simulink model "LundellAlternatorAC"  (R2018a)
settings: Solver=VariableStepAuto  StartTime=0  StopTime=0.2  FixedStep=1e-6
undefined symbols (not defined in the file): alternator, i_f, n_r, r_l
libraries: fl_lib x28, nesl_utility x27, powerlib_meascontrol x6, elec_lib x6, SimscapeCustomBlocks_lib x2
settings Model: Creator=gabrielrodrigues  LastModifiedBy=gabrielrodrigues
settings DataIOCC: ReturnWorkspaceOutputs=on
settings CodeAppCC: StateflowObjectComments=on
settings SimscapeCC: SimscapeNormalizeSystem=off  SimscapeLogType=local  SimscapeLogLimitData=off

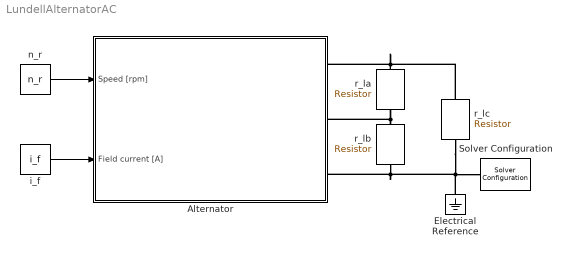
== system LundellAlternatorAC ==
  Alternator : Subsystem
  Electrical Reference : fl_lib/Electrical/Electrical Elements/Electrical Reference
  Solver Configuration : nesl_utility/Solver Configuration  PhysicalDomain=network_engine_domain  SubClassName=solver  LeftPortType=input  RightPortType=generic  Tones=[]  Harmonics=[]  SimulateNoise=off  Profile=off  UseLocalSampling=off  EnableSwitchedLinearOptims=on  FrequencyDomain=off  UseCCode=off  RelTol=0.001  AbsTol=1e-06  MinStep=1e-09  ToWorkspace=off  RevertToSquareIcSolve=off  NumHomotopyIterations=100  PhasorMode=off  PhasorModeNumHarmonics=1  DoDC=off  ResidualTolerance=1e-09  UseLocalSolver=on  LocalSolverChoice=NE_TRAPEZOIDAL_ADVANCER  LocalSolverSampleTime=1e-06  DoFixedCost=on  MaxNonlinIter=20  MaxModeIter=2  LinearAlgebra=Sparse  EquationFormulation=NE_TIME_EF  DelaysMemoryBudget=1024  AutomaticFiltering=on  FilteringTimeConstant=0.001
  i_f : Constant  Value=i_f
  n_r : Constant  Value=n_r
  r_la : fl_lib/Electrical/Electrical Elements/Resistor  R=r_l Ohm  i_specify=off  i_priority=None  i=0 A  i_nominal_specify=off  i_nominal_unit=A  i_nominal_value=1  v_specify=off  v_priority=None  v=0 V  v_nominal_specify=off  v_nominal_unit=V  v_nominal_value=1
  r_lb : fl_lib/Electrical/Electrical Elements/Resistor  R=r_l Ohm  i_specify=off  i_priority=None  i=0 A  i_nominal_specify=off  i_nominal_unit=A  i_nominal_value=1  v_specify=off  v_priority=None  v=0 V  v_nominal_specify=off  v_nominal_unit=V  v_nominal_value=1
  r_lc : fl_lib/Electrical/Electrical Elements/Resistor  R=r_l Ohm  i_specify=off  i_priority=None  i=0 A  i_nominal_specify=off  i_nominal_unit=A  i_nominal_value=1  v_specify=off  v_priority=None  v=0 V  v_nominal_specify=off  v_nominal_unit=V  v_nominal_value=1
  wires:
  n_r/1 -> Alternator/1(Speed [rpm])
  i_f/1 -> Alternator/2(Field current [A])
  connections:
  r_la/RConn1 -- r_lb/LConn1 -- Alternator/RConn2
  Electrical Reference/LConn1 -- Solver Configuration/RConn1 -- Alternator/RConn3 -- r_lb/RConn1 -- r_lc/LConn1
  r_la/LConn1 -- r_lc/RConn1 -- Alternator/RConn1

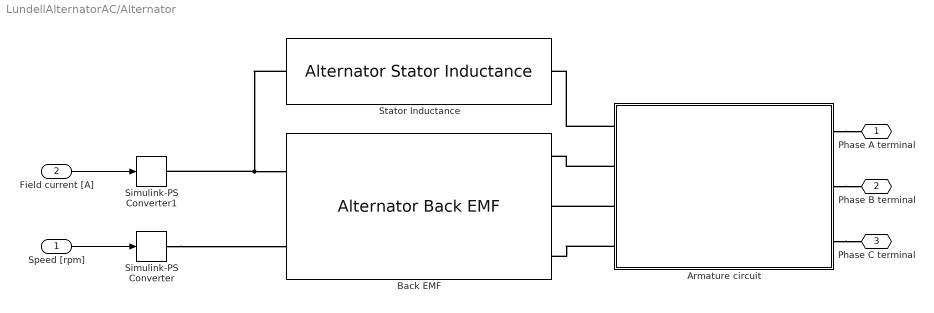
== system LundellAlternatorAC/Alternator ==
  Speed [rpm] : Inport
  Field current [A] : Inport  Port=2
  Armature circuit : Subsystem  Variant=on
  Back EMF : SimscapeCustomBlocks_lib/Alternator/Alternator Back EMF  p=alternator.p  omega_r_specify=off  omega_r_priority=None  omega_r=0 rad/s  omega_r_nominal_specify=off  omega_r_nominal_unit=rad/s  omega_r_nominal_value=1  omega_e_specify=off  omega_e_priority=None  omega_e=0 rad/s  omega_e_nominal_specify=off  omega_e_nominal_unit=rad/s  omega_e_nominal_value=1  theta_e_specify=off  theta_e_priority=None  theta_e=0 rad  theta_e_nominal_specify=off  theta_e_nominal_unit=rad  theta_e_nominal_value=1  k_e_specify=off  k_e_priority=None  k_e=0 s*V/rad/A  k_e_nominal_specify=off  k_e_nominal_unit=s*V/rad/A  k_e_nominal_value=1  e_specify=off  e_priority=None  e=0 rpm  e_nominal_specify=off  e_nominal_unit=rpm  e_nominal_value=1
  Simulink-PS Converter : nesl_utility/Simulink-PS Converter  PhysicalDomain=network_engine_domain  SubClassName=ps_input  LeftPortType=input  RightPortType=output  PseudoPeriodic=off  Frequencies=[]  NoiseDistribution=none  NoiseParameters=[]  Unit=1  AffineConversion=off  FilteringAndDerivatives=provide  SimscapeFilterOrder=1  InputFilterTimeConstant=0.001  UdotUserProvided=0
  Simulink-PS Converter1 : nesl_utility/Simulink-PS Converter  PhysicalDomain=network_engine_domain  SubClassName=ps_input  LeftPortType=input  RightPortType=output  PseudoPeriodic=off  Frequencies=[]  NoiseDistribution=none  NoiseParameters=[]  Unit=1  AffineConversion=off  FilteringAndDerivatives=provide  SimscapeFilterOrder=1  InputFilterTimeConstant=0.001  UdotUserProvided=0
  Stator Inductance : SimscapeCustomBlocks_lib/Alternator/Alternator Stator Inductance
  Phase A terminal : PMIOPort  Side=Right
  Phase B terminal : PMIOPort  Port=2  Side=Right
  Phase C terminal : PMIOPort  Port=3  Side=Right
  wires:
  Speed [rpm]/1 -> Simulink-PS Converter/1
  Field current [A]/1 -> Simulink-PS Converter1/1
  connections:
  Armature circuit/RConn1 -- Phase A terminal/RConn1
  Armature circuit/RConn2 -- Phase B terminal/RConn1
  Armature circuit/RConn3 -- Phase C terminal/RConn1
  Armature circuit/LConn3 -- Back EMF/RConn2
  Armature circuit/LConn2 -- Back EMF/RConn1
  Armature circuit/LConn4 -- Back EMF/RConn3
  Simulink-PS Converter/RConn1 -- Back EMF/LConn2
  Armature circuit/LConn1 -- Stator Inductance/RConn1
  Stator Inductance/LConn1 -- Simulink-PS Converter1/RConn1 -- Back EMF/LConn1

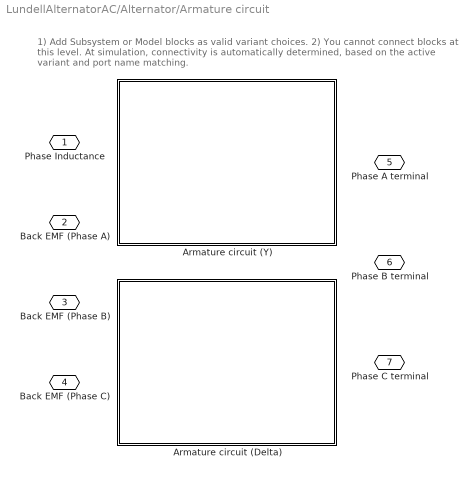
== system LundellAlternatorAC/Alternator/Armature circuit ==
  note: 1) Add Subsystem or Model blocks as valid variant choices.
      | 2) You cannot connect blocks at this level. At simulation, connectivity is automatically
      | determined, based on the active variant and port name matching.
  Armature circuit (Delta) : Subsystem  VariantControl=deltaStatorConnection
  Armature circuit (Y) : Subsystem  VariantControl=yStatorConnection
  Phase Inductance : PMIOPort  Side=Left
  Back EMF (Phase A) : PMIOPort  Port=2  Side=Left
  Back EMF (Phase B) : PMIOPort  Port=3  Side=Left
  Back EMF (Phase C) : PMIOPort  Port=4  Side=Left
  Phase A terminal : PMIOPort  Port=5  Side=Right
  Phase B terminal : PMIOPort  Port=6  Side=Right
  Phase C terminal : PMIOPort  Port=7  Side=Right

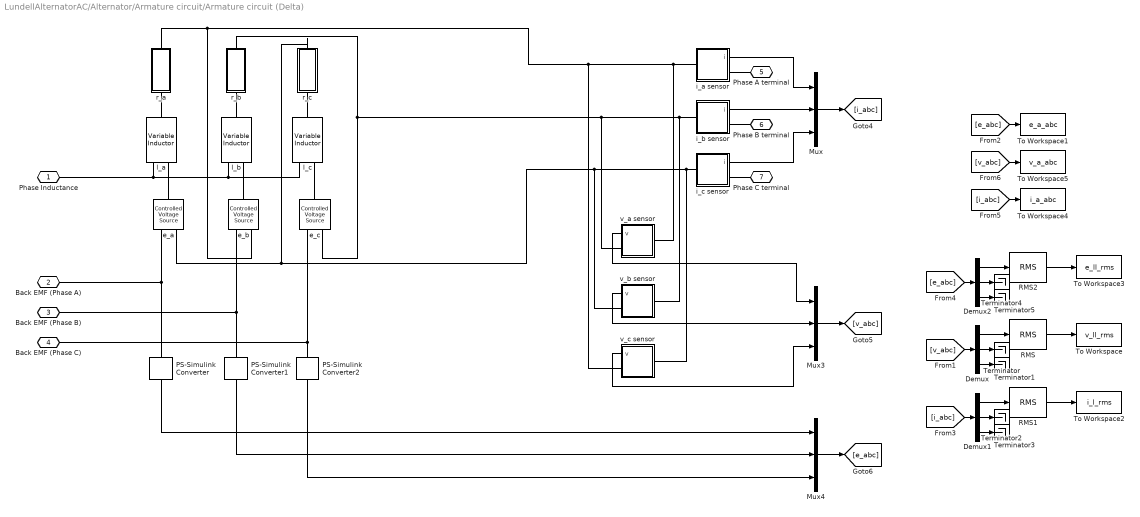
== system LundellAlternatorAC/Alternator/Armature circuit/Armature circuit (Delta) ==
  Demux : Demux  Outputs=3
  Demux1 : Demux  Outputs=3
  Demux2 : Demux  Outputs=3
  Mux : Mux  Inputs=3
  Mux3 : Mux  Inputs=3
  Mux4 : Mux  Inputs=3
  PS-Simulink Converter : nesl_utility/PS-Simulink Converter  PhysicalDomain=network_engine_domain  SubClassName=ps_output  LeftPortType=input  RightPortType=output  PseudoPeriodic=off  Frequencies=[]  Unit=1  AffineConversion=off
  PS-Simulink Converter1 : nesl_utility/PS-Simulink Converter  PhysicalDomain=network_engine_domain  SubClassName=ps_output  LeftPortType=input  RightPortType=output  PseudoPeriodic=off  Frequencies=[]  Unit=1  AffineConversion=off
  PS-Simulink Converter2 : nesl_utility/PS-Simulink Converter  PhysicalDomain=network_engine_domain  SubClassName=ps_output  LeftPortType=input  RightPortType=output  PseudoPeriodic=off  Frequencies=[]  Unit=1  AffineConversion=off
  RMS : powerlib_meascontrol/Measurements/RMS  TrueRMS=on  Freq=8*2000/60  RMSInit=120  Ts=0
      settings: SourceProductName=Simscape Electrical
  RMS1 : powerlib_meascontrol/Measurements/RMS  TrueRMS=on  Freq=8*2000/60  RMSInit=120  Ts=0
      settings: SourceProductName=Simscape Electrical
  RMS2 : powerlib_meascontrol/Measurements/RMS  TrueRMS=on  Freq=8*2000/60  RMSInit=120  Ts=0
      settings: SourceProductName=Simscape Electrical
  Terminator{,1..5} (6 alike) : Terminator
  To Workspace : ToWorkspace  VariableName=v_ll_rms  SaveFormat=Timeseries  SampleTime=-1
  To Workspace1 : ToWorkspace  VariableName=e_a_abc  SaveFormat=Timeseries  SampleTime=-1
  To Workspace2 : ToWorkspace  VariableName=i_l_rms  SaveFormat=Timeseries  SampleTime=-1
  To Workspace3 : ToWorkspace  VariableName=e_ll_rms  SaveFormat=Timeseries  SampleTime=-1
  To Workspace4 : ToWorkspace  VariableName=i_a_abc  SaveFormat=Timeseries  SampleTime=-1
  To Workspace5 : ToWorkspace  VariableName=v_a_abc  SaveFormat=Timeseries  SampleTime=-1
  e_a : fl_lib/Electrical/Electrical Sources/Controlled Voltage Source
  e_b : fl_lib/Electrical/Electrical Sources/Controlled Voltage Source
  e_c : fl_lib/Electrical/Electrical Sources/Controlled Voltage Source
  i_a sensor : Subsystem
  i_b sensor : Subsystem
  i_c sensor : Subsystem
  l_a : elec_lib/Passive Devices/Variable Inductor  prm=1  Lmin=1e-6 H  g=1e-9 1/Ohm  i0=0 A  phi0=0 Wb
      settings: SourceProductName=Simscape Electronics  SourceProductBaseCode=SN
  l_b : elec_lib/Passive Devices/Variable Inductor  prm=1  Lmin=1e-6 H  g=1e-9 1/Ohm  i0=0 A  phi0=0 Wb
      settings: SourceProductName=Simscape Electronics  SourceProductBaseCode=SN
  l_c : elec_lib/Passive Devices/Variable Inductor  prm=1  Lmin=1e-6 H  g=1e-9 1/Ohm  i0=0 A  phi0=0 Wb
      settings: SourceProductName=Simscape Electronics  SourceProductBaseCode=SN
  r_a : Subsystem  mask{r_ref=alternator.stator.r.value, T_ref=alternator.stator.r.T_ref, T=alternator.stator.r.T, alpha=alternator.stator.r.alpha}
      mask prompts: r_ref "Nominal resistance [Ohm]"; T_ref "Reference temperature [oC]"; T "Resistor temperature [oC]"; alpha "Temperature Coefficient [1/oC]"
  r_b : Subsystem  mask{r_ref=alternator.stator.r.value, T_ref=alternator.stator.r.T_ref, T=alternator.stator.r.T, alpha=alternator.stator.r.alpha}
      mask prompts: r_ref "Nominal resistance [Ohm]"; T_ref "Reference temperature [oC]"; T "Resistor temperature [oC]"; alpha "Temperature Coefficient [1/oC]"
  r_c : Subsystem  mask{r_ref=alternator.stator.r.value, T_ref=alternator.stator.r.T_ref, T=alternator.stator.r.T, alpha=alternator.stator.r.alpha}
      mask prompts: r_ref "Nominal resistance [Ohm]"; T_ref "Reference temperature [oC]"; T "Resistor temperature [oC]"; alpha "Temperature Coefficient [1/oC]"
  v_a sensor : Subsystem
  v_b sensor : Subsystem
  v_c sensor : Subsystem
  Phase Inductance : PMIOPort  Side=Left
  Back EMF (Phase A) : PMIOPort  Port=2  Side=Left
  Back EMF (Phase B) : PMIOPort  Port=3  Side=Left
  Back EMF (Phase C) : PMIOPort  Port=4  Side=Left
  Phase A terminal : PMIOPort  Port=5  Side=Right
  Phase B terminal : PMIOPort  Port=6  Side=Right
  Phase C terminal : PMIOPort  Port=7  Side=Right
  wires:
  i_a sensor/1(i) -> Mux/1
  i_b sensor/1(i) -> Mux/2
  i_c sensor/1(i) -> Mux/3
  Mux/1 -> [i_abc]
  Mux3/1 -> [v_abc]
  v_b sensor/1(v) -> Mux3/2
  v_c sensor/1(v) -> Mux3/3
  v_a sensor/1(v) -> Mux3/1
  PS-Simulink Converter/1 -> Mux4/1
  PS-Simulink Converter1/1 -> Mux4/2
  PS-Simulink Converter2/1 -> Mux4/3
  Mux4/1 -> [e_abc]
  Demux/3 -> Terminator1/1
  Demux/2 -> Terminator/1
  Demux2/2 -> Terminator4/1
  [e_abc] -> Demux2/1
  RMS2/1 -> To Workspace3/1
  Demux2/1 -> RMS2/1
  Demux2/3 -> Terminator5/1
  Demux1/2 -> Terminator2/1
  [e_abc] -> To Workspace1/1
  RMS/1 -> To Workspace/1
  Demux/1 -> RMS/1
  RMS1/1 -> To Workspace2/1
  [i_abc] -> Demux1/1
  [v_abc] -> Demux/1
  Demux1/3 -> Terminator3/1
  [v_abc] -> To Workspace5/1
  Demux1/1 -> RMS1/1
  [i_abc] -> To Workspace4/1
  connections:
  i_a sensor/RConn1 -- Phase A terminal/RConn1
  Back EMF (Phase A)/RConn1 -- e_a/RConn1 -- PS-Simulink Converter/LConn1
  Back EMF (Phase B)/RConn1 -- e_b/RConn1 -- PS-Simulink Converter1/LConn1
  Back EMF (Phase C)/RConn1 -- e_c/RConn1 -- PS-Simulink Converter2/LConn1
  e_c/LConn1 -- l_c/LConn2
  e_b/LConn1 -- l_b/LConn2
  e_a/LConn1 -- l_a/LConn2
  r_c/LConn1 -- l_c/RConn1
  r_b/LConn1 -- l_b/RConn1
  r_a/LConn1 -- l_a/RConn1
  i_c sensor/RConn1 -- Phase C terminal/RConn1
  i_b sensor/RConn1 -- Phase B terminal/RConn1
  l_a/LConn1 -- Phase Inductance/RConn1 -- l_b/LConn1 -- l_c/LConn1
  e_b/RConn2 -- v_a sensor/LConn1 -- i_a sensor/LConn1 -- v_c sensor/RConn1 -- r_a/RConn1
  v_a sensor/RConn1 -- i_b sensor/LConn1 -- v_b sensor/LConn1 -- e_c/RConn2 -- r_b/RConn1
  e_a/RConn2 -- v_c sensor/LConn1 -- i_c sensor/LConn1 -- v_b sensor/RConn1 -- r_c/RConn1

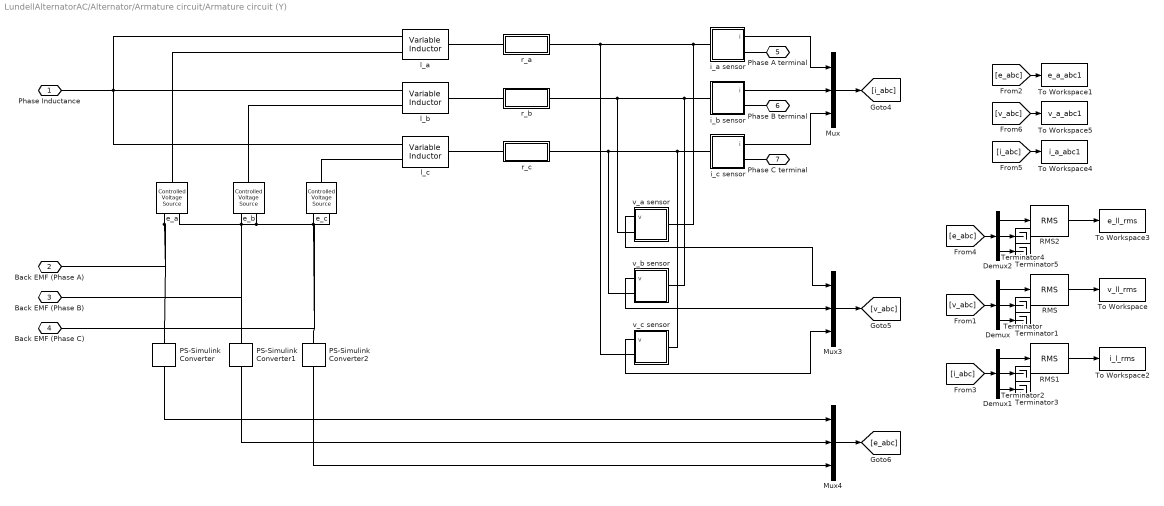
== system LundellAlternatorAC/Alternator/Armature circuit/Armature circuit (Y) ==
  Demux : Demux  Outputs=3
  Demux1 : Demux  Outputs=3
  Demux2 : Demux  Outputs=3
  Mux : Mux  Inputs=3
  Mux3 : Mux  Inputs=3
  Mux4 : Mux  Inputs=3
  PS-Simulink Converter : nesl_utility/PS-Simulink Converter  PhysicalDomain=network_engine_domain  SubClassName=ps_output  LeftPortType=input  RightPortType=output  PseudoPeriodic=off  Frequencies=[]  Unit=1  AffineConversion=off
  PS-Simulink Converter1 : nesl_utility/PS-Simulink Converter  PhysicalDomain=network_engine_domain  SubClassName=ps_output  LeftPortType=input  RightPortType=output  PseudoPeriodic=off  Frequencies=[]  Unit=1  AffineConversion=off
  PS-Simulink Converter2 : nesl_utility/PS-Simulink Converter  PhysicalDomain=network_engine_domain  SubClassName=ps_output  LeftPortType=input  RightPortType=output  PseudoPeriodic=off  Frequencies=[]  Unit=1  AffineConversion=off
  RMS : powerlib_meascontrol/Measurements/RMS  TrueRMS=on  Freq=8*2000/60  RMSInit=120  Ts=0
      settings: SourceProductName=Simscape Electrical
  RMS1 : powerlib_meascontrol/Measurements/RMS  TrueRMS=on  Freq=8*2000/60  RMSInit=120  Ts=0
      settings: SourceProductName=Simscape Electrical
  RMS2 : powerlib_meascontrol/Measurements/RMS  TrueRMS=on  Freq=8*2000/60  RMSInit=120  Ts=0
      settings: SourceProductName=Simscape Electrical
  Terminator{,1..5} (6 alike) : Terminator
  To Workspace : ToWorkspace  VariableName=v_ll_rms  SaveFormat=Timeseries  SampleTime=-1
  To Workspace1 : ToWorkspace  VariableName=e_a_abc1  SaveFormat=Timeseries  SampleTime=-1
  To Workspace2 : ToWorkspace  VariableName=i_l_rms  SaveFormat=Timeseries  SampleTime=-1
  To Workspace3 : ToWorkspace  VariableName=e_ll_rms  SaveFormat=Timeseries  SampleTime=-1
  To Workspace4 : ToWorkspace  VariableName=i_a_abc1  SaveFormat=Timeseries  SampleTime=-1
  To Workspace5 : ToWorkspace  VariableName=v_a_abc1  SaveFormat=Timeseries  SampleTime=-1
  e_a : fl_lib/Electrical/Electrical Sources/Controlled Voltage Source
  e_b : fl_lib/Electrical/Electrical Sources/Controlled Voltage Source
  e_c : fl_lib/Electrical/Electrical Sources/Controlled Voltage Source
  i_a sensor : Subsystem
  i_b sensor : Subsystem
  i_c sensor : Subsystem
  l_a : elec_lib/Passive Devices/Variable Inductor  prm=1  Lmin=1e-6 H  g=1e-9 1/Ohm  i0=0 A  phi0=0 Wb
      settings: SourceProductName=Simscape Electronics  SourceProductBaseCode=SN
  l_b : elec_lib/Passive Devices/Variable Inductor  prm=1  Lmin=1e-6 H  g=1e-9 1/Ohm  i0=0 A  phi0=0 Wb
      settings: SourceProductName=Simscape Electronics  SourceProductBaseCode=SN
  l_c : elec_lib/Passive Devices/Variable Inductor  prm=1  Lmin=1e-6 H  g=1e-9 1/Ohm  i0=0 A  phi0=0 Wb
      settings: SourceProductName=Simscape Electronics  SourceProductBaseCode=SN
  r_a : Subsystem  mask{r_ref=alternator.stator.r.value, T_ref=alternator.stator.r.T_ref, T=alternator.stator.r.T, alpha=alternator.stator.r.alpha}
      mask prompts: r_ref "Nominal resistance [Ohm]"; T_ref "Reference temperature [oC]"; T "Resistor temperature [oC]"; alpha "Temperature Coefficient [1/oC]"
  r_b : Subsystem  mask{r_ref=alternator.stator.r.value, T_ref=alternator.stator.r.T_ref, T=alternator.stator.r.T, alpha=alternator.stator.r.alpha}
      mask prompts: r_ref "Nominal resistance [Ohm]"; T_ref "Reference temperature [oC]"; T "Resistor temperature [oC]"; alpha "Temperature Coefficient [1/oC]"
  r_c : Subsystem  mask{r_ref=alternator.stator.r.value, T_ref=alternator.stator.r.T_ref, T=alternator.stator.r.T, alpha=alternator.stator.r.alpha}
      mask prompts: r_ref "Nominal resistance [Ohm]"; T_ref "Reference temperature [oC]"; T "Resistor temperature [oC]"; alpha "Temperature Coefficient [1/oC]"
  v_a sensor : Subsystem
  v_b sensor : Subsystem
  v_c sensor : Subsystem
  Phase Inductance : PMIOPort  Side=Left
  Back EMF (Phase A) : PMIOPort  Port=2  Side=Left
  Back EMF (Phase B) : PMIOPort  Port=3  Side=Left
  Back EMF (Phase C) : PMIOPort  Port=4  Side=Left
  Phase A terminal : PMIOPort  Port=5  Side=Right
  Phase B terminal : PMIOPort  Port=6  Side=Right
  Phase C terminal : PMIOPort  Port=7  Side=Right
  wires:
  i_a sensor/1(i) -> Mux/1
  i_b sensor/1(i) -> Mux/2
  i_c sensor/1(i) -> Mux/3
  Mux/1 -> [i_abc]
  Mux3/1 -> [v_abc]
  v_b sensor/1(v) -> Mux3/2
  v_c sensor/1(v) -> Mux3/3
  v_a sensor/1(v) -> Mux3/1
  PS-Simulink Converter/1 -> Mux4/1
  PS-Simulink Converter1/1 -> Mux4/2
  PS-Simulink Converter2/1 -> Mux4/3
  Mux4/1 -> [e_abc]
  Demux/3 -> Terminator1/1
  Demux/2 -> Terminator/1
  Demux2/2 -> Terminator4/1
  [e_abc] -> Demux2/1
  RMS2/1 -> To Workspace3/1
  Demux2/1 -> RMS2/1
  Demux2/3 -> Terminator5/1
  Demux1/2 -> Terminator2/1
  [e_abc] -> To Workspace1/1
  RMS/1 -> To Workspace/1
  Demux/1 -> RMS/1
  RMS1/1 -> To Workspace2/1
  [i_abc] -> Demux1/1
  [v_abc] -> Demux/1
  Demux1/3 -> Terminator3/1
  [v_abc] -> To Workspace5/1
  Demux1/1 -> RMS1/1
  [i_abc] -> To Workspace4/1
  connections:
  i_a sensor/RConn1 -- Phase A terminal/RConn1
  e_a/RConn2 -- e_c/RConn2 -- e_b/RConn2
  e_c/LConn1 -- l_c/LConn2
  e_b/LConn1 -- l_b/LConn2
  e_a/LConn1 -- l_a/LConn2
  r_c/LConn1 -- l_c/RConn1
  r_b/LConn1 -- l_b/RConn1
  r_a/LConn1 -- l_a/RConn1
  i_a sensor/LConn1 -- v_a sensor/LConn1 -- v_c sensor/RConn1 -- r_a/RConn1
  i_c sensor/RConn1 -- Phase C terminal/RConn1
  i_b sensor/RConn1 -- Phase B terminal/RConn1
  i_c sensor/LConn1 -- v_c sensor/LConn1 -- v_b sensor/RConn1 -- r_c/RConn1
  v_a sensor/RConn1 -- v_b sensor/LConn1 -- i_b sensor/LConn1 -- r_b/RConn1
  l_a/LConn1 -- Phase Inductance/RConn1 -- l_c/LConn1 -- l_b/LConn1
  e_a/RConn1 -- Back EMF (Phase A)/RConn1 -- PS-Simulink Converter/LConn1
  e_b/RConn1 -- Back EMF (Phase B)/RConn1 -- PS-Simulink Converter1/LConn1
  e_c/RConn1 -- Back EMF (Phase C)/RConn1 -- PS-Simulink Converter2/LConn1

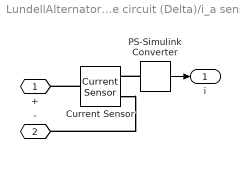
== system LundellAlternatorAC/Alternator/Armature circuit/Armature circuit (Delta)/i_a sensor ==
  Current Sensor : fl_lib/Electrical/Electrical Sensors/Current Sensor
  PS-Simulink Converter : nesl_utility/PS-Simulink Converter  PhysicalDomain=network_engine_domain  SubClassName=ps_output  LeftPortType=input  RightPortType=output  PseudoPeriodic=off  Frequencies=[]  Unit=1  AffineConversion=off
  + : PMIOPort  Side=Left
  - : PMIOPort  Port=2  Side=Right
  i : Outport
  wires:
  PS-Simulink Converter/1 -> i/1
  connections:
  Current Sensor/RConn2 -- -/RConn1
  Current Sensor/LConn1 -- +/RConn1
  PS-Simulink Converter/LConn1 -- Current Sensor/RConn1

== system LundellAlternatorAC/Alternator/Armature circuit/Armature circuit (Delta)/i_b sensor ==
  Current Sensor : fl_lib/Electrical/Electrical Sensors/Current Sensor
  PS-Simulink Converter : nesl_utility/PS-Simulink Converter  PhysicalDomain=network_engine_domain  SubClassName=ps_output  LeftPortType=input  RightPortType=output  PseudoPeriodic=off  Frequencies=[]  Unit=1  AffineConversion=off
  + : PMIOPort  Side=Left
  - : PMIOPort  Port=2  Side=Right
  i : Outport
  wires:
  PS-Simulink Converter/1 -> i/1
  connections:
  Current Sensor/RConn2 -- -/RConn1
  Current Sensor/LConn1 -- +/RConn1
  PS-Simulink Converter/LConn1 -- Current Sensor/RConn1

== system LundellAlternatorAC/Alternator/Armature circuit/Armature circuit (Delta)/i_c sensor ==
  Current Sensor : fl_lib/Electrical/Electrical Sensors/Current Sensor
  PS-Simulink Converter : nesl_utility/PS-Simulink Converter  PhysicalDomain=network_engine_domain  SubClassName=ps_output  LeftPortType=input  RightPortType=output  PseudoPeriodic=off  Frequencies=[]  Unit=1  AffineConversion=off
  + : PMIOPort  Side=Left
  - : PMIOPort  Port=2  Side=Right
  i : Outport
  wires:
  PS-Simulink Converter/1 -> i/1
  connections:
  Current Sensor/RConn2 -- -/RConn1
  Current Sensor/LConn1 -- +/RConn1
  PS-Simulink Converter/LConn1 -- Current Sensor/RConn1

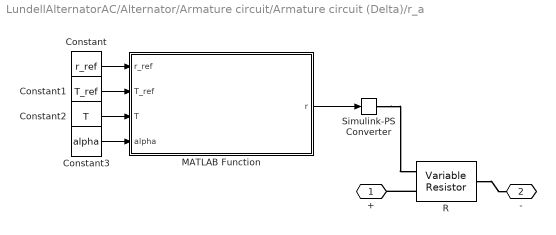
== system LundellAlternatorAC/Alternator/Armature circuit/Armature circuit (Delta)/r_a ==
  Constant : Constant  Value=r_ref
  Constant1 : Constant  Value=T_ref
  Constant2 : Constant  Value=T
  Constant3 : Constant  Value=alpha
  MATLAB Function : MATLAB Function  TreatAsAtomicUnit=on
  R : fl_lib/Electrical/Electrical Elements/Variable Resistor  Rmin=0 Ohm  i_specify=off  i_priority=None  i=0 A  i_nominal_specify=off  i_nominal_unit=A  i_nominal_value=1  v_specify=off  v_priority=None  v=0 V  v_nominal_specify=off  v_nominal_unit=V  v_nominal_value=1
  Simulink-PS Converter : nesl_utility/Simulink-PS Converter  PhysicalDomain=network_engine_domain  SubClassName=ps_input  LeftPortType=input  RightPortType=output  PseudoPeriodic=off  Frequencies=[]  NoiseDistribution=none  NoiseParameters=[]  Unit=1  AffineConversion=off  FilteringAndDerivatives=provide  SimscapeFilterOrder=1  InputFilterTimeConstant=0.001  UdotUserProvided=0
  + : PMIOPort  Side=Left
  - : PMIOPort  Port=2  Side=Right
  wires:
  MATLAB Function/1(r) -> Simulink-PS Converter/1
  Constant/1 -> MATLAB Function/1(r_ref)
  Constant1/1 -> MATLAB Function/2(T_ref)
  Constant3/1 -> MATLAB Function/4(alpha)
  Constant2/1 -> MATLAB Function/3(T)
  connections:
  Simulink-PS Converter/RConn1 -- R/LConn1
  R/RConn1 -- -/RConn1
  R/LConn2 -- +/RConn1

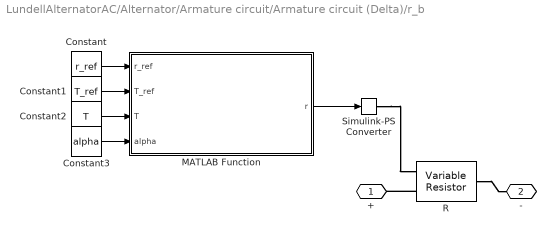
== system LundellAlternatorAC/Alternator/Armature circuit/Armature circuit (Delta)/r_b ==
  Constant : Constant  Value=r_ref
  Constant1 : Constant  Value=T_ref
  Constant2 : Constant  Value=T
  Constant3 : Constant  Value=alpha
  MATLAB Function : MATLAB Function  TreatAsAtomicUnit=on
  R : fl_lib/Electrical/Electrical Elements/Variable Resistor  Rmin=0 Ohm  i_specify=off  i_priority=None  i=0 A  i_nominal_specify=off  i_nominal_unit=A  i_nominal_value=1  v_specify=off  v_priority=None  v=0 V  v_nominal_specify=off  v_nominal_unit=V  v_nominal_value=1
  Simulink-PS Converter : nesl_utility/Simulink-PS Converter  PhysicalDomain=network_engine_domain  SubClassName=ps_input  LeftPortType=input  RightPortType=output  PseudoPeriodic=off  Frequencies=[]  NoiseDistribution=none  NoiseParameters=[]  Unit=1  AffineConversion=off  FilteringAndDerivatives=provide  SimscapeFilterOrder=1  InputFilterTimeConstant=0.001  UdotUserProvided=0
  + : PMIOPort  Side=Left
  - : PMIOPort  Port=2  Side=Right
  wires:
  MATLAB Function/1(r) -> Simulink-PS Converter/1
  Constant/1 -> MATLAB Function/1(r_ref)
  Constant1/1 -> MATLAB Function/2(T_ref)
  Constant3/1 -> MATLAB Function/4(alpha)
  Constant2/1 -> MATLAB Function/3(T)
  connections:
  Simulink-PS Converter/RConn1 -- R/LConn1
  R/RConn1 -- -/RConn1
  R/LConn2 -- +/RConn1

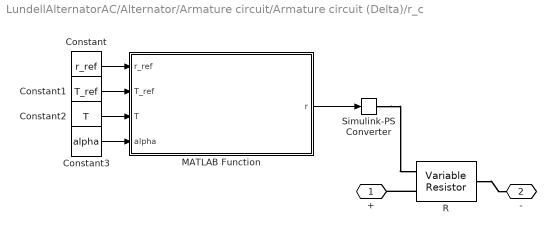
== system LundellAlternatorAC/Alternator/Armature circuit/Armature circuit (Delta)/r_c ==
  Constant : Constant  Value=r_ref
  Constant1 : Constant  Value=T_ref
  Constant2 : Constant  Value=T
  Constant3 : Constant  Value=alpha
  MATLAB Function : MATLAB Function  TreatAsAtomicUnit=on
  R : fl_lib/Electrical/Electrical Elements/Variable Resistor  Rmin=0 Ohm  i_specify=off  i_priority=None  i=0 A  i_nominal_specify=off  i_nominal_unit=A  i_nominal_value=1  v_specify=off  v_priority=None  v=0 V  v_nominal_specify=off  v_nominal_unit=V  v_nominal_value=1
  Simulink-PS Converter : nesl_utility/Simulink-PS Converter  PhysicalDomain=network_engine_domain  SubClassName=ps_input  LeftPortType=input  RightPortType=output  PseudoPeriodic=off  Frequencies=[]  NoiseDistribution=none  NoiseParameters=[]  Unit=1  AffineConversion=off  FilteringAndDerivatives=provide  SimscapeFilterOrder=1  InputFilterTimeConstant=0.001  UdotUserProvided=0
  + : PMIOPort  Side=Left
  - : PMIOPort  Port=2  Side=Right
  wires:
  MATLAB Function/1(r) -> Simulink-PS Converter/1
  Constant/1 -> MATLAB Function/1(r_ref)
  Constant1/1 -> MATLAB Function/2(T_ref)
  Constant3/1 -> MATLAB Function/4(alpha)
  Constant2/1 -> MATLAB Function/3(T)
  connections:
  Simulink-PS Converter/RConn1 -- R/LConn1
  R/RConn1 -- -/RConn1
  R/LConn2 -- +/RConn1

== system LundellAlternatorAC/Alternator/Armature circuit/Armature circuit (Delta)/v_a sensor ==
  PS-Simulink Converter : nesl_utility/PS-Simulink Converter  PhysicalDomain=network_engine_domain  SubClassName=ps_output  LeftPortType=input  RightPortType=output  PseudoPeriodic=off  Frequencies=[]  Unit=1  AffineConversion=off
  Voltage Sensor : fl_lib/Electrical/Electrical Sensors/Voltage Sensor
  + : PMIOPort  Side=Left
  - : PMIOPort  Port=2  Side=Right
  v : Outport
  wires:
  PS-Simulink Converter/1 -> v/1
  connections:
  Voltage Sensor/LConn1 -- +/RConn1
  -/RConn1 -- Voltage Sensor/RConn2
  Voltage Sensor/RConn1 -- PS-Simulink Converter/LConn1

== system LundellAlternatorAC/Alternator/Armature circuit/Armature circuit (Delta)/v_b sensor ==
  PS-Simulink Converter : nesl_utility/PS-Simulink Converter  PhysicalDomain=network_engine_domain  SubClassName=ps_output  LeftPortType=input  RightPortType=output  PseudoPeriodic=off  Frequencies=[]  Unit=1  AffineConversion=off
  Voltage Sensor : fl_lib/Electrical/Electrical Sensors/Voltage Sensor
  + : PMIOPort  Side=Left
  - : PMIOPort  Port=2  Side=Right
  v : Outport
  wires:
  PS-Simulink Converter/1 -> v/1
  connections:
  Voltage Sensor/LConn1 -- +/RConn1
  -/RConn1 -- Voltage Sensor/RConn2
  Voltage Sensor/RConn1 -- PS-Simulink Converter/LConn1

== system LundellAlternatorAC/Alternator/Armature circuit/Armature circuit (Delta)/v_c sensor ==
  PS-Simulink Converter : nesl_utility/PS-Simulink Converter  PhysicalDomain=network_engine_domain  SubClassName=ps_output  LeftPortType=input  RightPortType=output  PseudoPeriodic=off  Frequencies=[]  Unit=1  AffineConversion=off
  Voltage Sensor : fl_lib/Electrical/Electrical Sensors/Voltage Sensor
  + : PMIOPort  Side=Left
  - : PMIOPort  Port=2  Side=Right
  v : Outport
  wires:
  PS-Simulink Converter/1 -> v/1
  connections:
  Voltage Sensor/LConn1 -- +/RConn1
  -/RConn1 -- Voltage Sensor/RConn2
  Voltage Sensor/RConn1 -- PS-Simulink Converter/LConn1

== system LundellAlternatorAC/Alternator/Armature circuit/Armature circuit (Y)/i_a sensor ==
  Current Sensor : fl_lib/Electrical/Electrical Sensors/Current Sensor
  PS-Simulink Converter : nesl_utility/PS-Simulink Converter  PhysicalDomain=network_engine_domain  SubClassName=ps_output  LeftPortType=input  RightPortType=output  PseudoPeriodic=off  Frequencies=[]  Unit=1  AffineConversion=off
  + : PMIOPort  Side=Left
  - : PMIOPort  Port=2  Side=Right
  i : Outport
  wires:
  PS-Simulink Converter/1 -> i/1
  connections:
  Current Sensor/RConn2 -- -/RConn1
  Current Sensor/LConn1 -- +/RConn1
  PS-Simulink Converter/LConn1 -- Current Sensor/RConn1

== system LundellAlternatorAC/Alternator/Armature circuit/Armature circuit (Y)/i_b sensor ==
  Current Sensor : fl_lib/Electrical/Electrical Sensors/Current Sensor
  PS-Simulink Converter : nesl_utility/PS-Simulink Converter  PhysicalDomain=network_engine_domain  SubClassName=ps_output  LeftPortType=input  RightPortType=output  PseudoPeriodic=off  Frequencies=[]  Unit=1  AffineConversion=off
  + : PMIOPort  Side=Left
  - : PMIOPort  Port=2  Side=Right
  i : Outport
  wires:
  PS-Simulink Converter/1 -> i/1
  connections:
  Current Sensor/RConn2 -- -/RConn1
  Current Sensor/LConn1 -- +/RConn1
  PS-Simulink Converter/LConn1 -- Current Sensor/RConn1

== system LundellAlternatorAC/Alternator/Armature circuit/Armature circuit (Y)/i_c sensor ==
  Current Sensor : fl_lib/Electrical/Electrical Sensors/Current Sensor
  PS-Simulink Converter : nesl_utility/PS-Simulink Converter  PhysicalDomain=network_engine_domain  SubClassName=ps_output  LeftPortType=input  RightPortType=output  PseudoPeriodic=off  Frequencies=[]  Unit=1  AffineConversion=off
  + : PMIOPort  Side=Left
  - : PMIOPort  Port=2  Side=Right
  i : Outport
  wires:
  PS-Simulink Converter/1 -> i/1
  connections:
  Current Sensor/RConn2 -- -/RConn1
  Current Sensor/LConn1 -- +/RConn1
  PS-Simulink Converter/LConn1 -- Current Sensor/RConn1

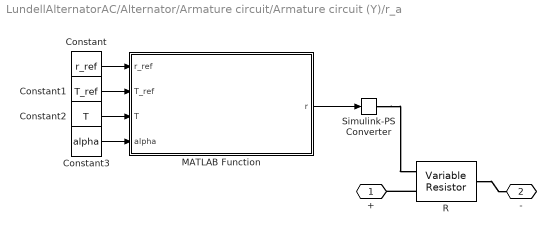
== system LundellAlternatorAC/Alternator/Armature circuit/Armature circuit (Y)/r_a ==
  Constant : Constant  Value=r_ref
  Constant1 : Constant  Value=T_ref
  Constant2 : Constant  Value=T
  Constant3 : Constant  Value=alpha
  MATLAB Function : MATLAB Function  TreatAsAtomicUnit=on
  R : fl_lib/Electrical/Electrical Elements/Variable Resistor  Rmin=0 Ohm  i_specify=off  i_priority=None  i=0 A  i_nominal_specify=off  i_nominal_unit=A  i_nominal_value=1  v_specify=off  v_priority=None  v=0 V  v_nominal_specify=off  v_nominal_unit=V  v_nominal_value=1
  Simulink-PS Converter : nesl_utility/Simulink-PS Converter  PhysicalDomain=network_engine_domain  SubClassName=ps_input  LeftPortType=input  RightPortType=output  PseudoPeriodic=off  Frequencies=[]  NoiseDistribution=none  NoiseParameters=[]  Unit=1  AffineConversion=off  FilteringAndDerivatives=provide  SimscapeFilterOrder=1  InputFilterTimeConstant=0.001  UdotUserProvided=0
  + : PMIOPort  Side=Left
  - : PMIOPort  Port=2  Side=Right
  wires:
  MATLAB Function/1(r) -> Simulink-PS Converter/1
  Constant/1 -> MATLAB Function/1(r_ref)
  Constant1/1 -> MATLAB Function/2(T_ref)
  Constant3/1 -> MATLAB Function/4(alpha)
  Constant2/1 -> MATLAB Function/3(T)
  connections:
  Simulink-PS Converter/RConn1 -- R/LConn1
  R/RConn1 -- -/RConn1
  R/LConn2 -- +/RConn1

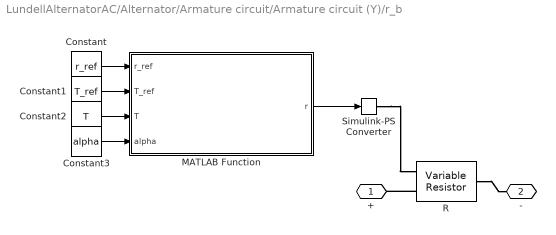
== system LundellAlternatorAC/Alternator/Armature circuit/Armature circuit (Y)/r_b ==
  Constant : Constant  Value=r_ref
  Constant1 : Constant  Value=T_ref
  Constant2 : Constant  Value=T
  Constant3 : Constant  Value=alpha
  MATLAB Function : MATLAB Function  TreatAsAtomicUnit=on
  R : fl_lib/Electrical/Electrical Elements/Variable Resistor  Rmin=0 Ohm  i_specify=off  i_priority=None  i=0 A  i_nominal_specify=off  i_nominal_unit=A  i_nominal_value=1  v_specify=off  v_priority=None  v=0 V  v_nominal_specify=off  v_nominal_unit=V  v_nominal_value=1
  Simulink-PS Converter : nesl_utility/Simulink-PS Converter  PhysicalDomain=network_engine_domain  SubClassName=ps_input  LeftPortType=input  RightPortType=output  PseudoPeriodic=off  Frequencies=[]  NoiseDistribution=none  NoiseParameters=[]  Unit=1  AffineConversion=off  FilteringAndDerivatives=provide  SimscapeFilterOrder=1  InputFilterTimeConstant=0.001  UdotUserProvided=0
  + : PMIOPort  Side=Left
  - : PMIOPort  Port=2  Side=Right
  wires:
  MATLAB Function/1(r) -> Simulink-PS Converter/1
  Constant/1 -> MATLAB Function/1(r_ref)
  Constant1/1 -> MATLAB Function/2(T_ref)
  Constant3/1 -> MATLAB Function/4(alpha)
  Constant2/1 -> MATLAB Function/3(T)
  connections:
  Simulink-PS Converter/RConn1 -- R/LConn1
  R/RConn1 -- -/RConn1
  R/LConn2 -- +/RConn1

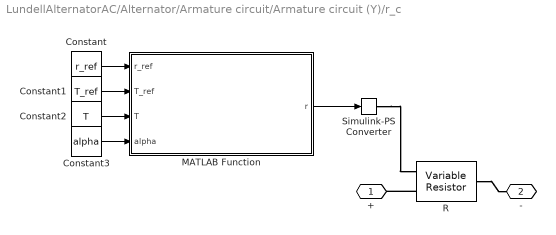
== system LundellAlternatorAC/Alternator/Armature circuit/Armature circuit (Y)/r_c ==
  Constant : Constant  Value=r_ref
  Constant1 : Constant  Value=T_ref
  Constant2 : Constant  Value=T
  Constant3 : Constant  Value=alpha
  MATLAB Function : MATLAB Function  TreatAsAtomicUnit=on
  R : fl_lib/Electrical/Electrical Elements/Variable Resistor  Rmin=0 Ohm  i_specify=off  i_priority=None  i=0 A  i_nominal_specify=off  i_nominal_unit=A  i_nominal_value=1  v_specify=off  v_priority=None  v=0 V  v_nominal_specify=off  v_nominal_unit=V  v_nominal_value=1
  Simulink-PS Converter : nesl_utility/Simulink-PS Converter  PhysicalDomain=network_engine_domain  SubClassName=ps_input  LeftPortType=input  RightPortType=output  PseudoPeriodic=off  Frequencies=[]  NoiseDistribution=none  NoiseParameters=[]  Unit=1  AffineConversion=off  FilteringAndDerivatives=provide  SimscapeFilterOrder=1  InputFilterTimeConstant=0.001  UdotUserProvided=0
  + : PMIOPort  Side=Left
  - : PMIOPort  Port=2  Side=Right
  wires:
  MATLAB Function/1(r) -> Simulink-PS Converter/1
  Constant/1 -> MATLAB Function/1(r_ref)
  Constant1/1 -> MATLAB Function/2(T_ref)
  Constant3/1 -> MATLAB Function/4(alpha)
  Constant2/1 -> MATLAB Function/3(T)
  connections:
  Simulink-PS Converter/RConn1 -- R/LConn1
  R/RConn1 -- -/RConn1
  R/LConn2 -- +/RConn1

== system LundellAlternatorAC/Alternator/Armature circuit/Armature circuit (Y)/v_a sensor ==
  PS-Simulink Converter : nesl_utility/PS-Simulink Converter  PhysicalDomain=network_engine_domain  SubClassName=ps_output  LeftPortType=input  RightPortType=output  PseudoPeriodic=off  Frequencies=[]  Unit=1  AffineConversion=off
  Voltage Sensor : fl_lib/Electrical/Electrical Sensors/Voltage Sensor
  + : PMIOPort  Side=Left
  - : PMIOPort  Port=2  Side=Right
  v : Outport
  wires:
  PS-Simulink Converter/1 -> v/1
  connections:
  Voltage Sensor/LConn1 -- +/RConn1
  -/RConn1 -- Voltage Sensor/RConn2
  Voltage Sensor/RConn1 -- PS-Simulink Converter/LConn1

== system LundellAlternatorAC/Alternator/Armature circuit/Armature circuit (Y)/v_b sensor ==
  PS-Simulink Converter : nesl_utility/PS-Simulink Converter  PhysicalDomain=network_engine_domain  SubClassName=ps_output  LeftPortType=input  RightPortType=output  PseudoPeriodic=off  Frequencies=[]  Unit=1  AffineConversion=off
  Voltage Sensor : fl_lib/Electrical/Electrical Sensors/Voltage Sensor
  + : PMIOPort  Side=Left
  - : PMIOPort  Port=2  Side=Right
  v : Outport
  wires:
  PS-Simulink Converter/1 -> v/1
  connections:
  Voltage Sensor/LConn1 -- +/RConn1
  -/RConn1 -- Voltage Sensor/RConn2
  Voltage Sensor/RConn1 -- PS-Simulink Converter/LConn1

== system LundellAlternatorAC/Alternator/Armature circuit/Armature circuit (Y)/v_c sensor ==
  PS-Simulink Converter : nesl_utility/PS-Simulink Converter  PhysicalDomain=network_engine_domain  SubClassName=ps_output  LeftPortType=input  RightPortType=output  PseudoPeriodic=off  Frequencies=[]  Unit=1  AffineConversion=off
  Voltage Sensor : fl_lib/Electrical/Electrical Sensors/Voltage Sensor
  + : PMIOPort  Side=Left
  - : PMIOPort  Port=2  Side=Right
  v : Outport
  wires:
  PS-Simulink Converter/1 -> v/1
  connections:
  Voltage Sensor/LConn1 -- +/RConn1
  -/RConn1 -- Voltage Sensor/RConn2
  Voltage Sensor/RConn1 -- PS-Simulink Converter/LConn1

== matlab function LundellAlternatorAC/Alternator/Armature circuit/Armature circuit (Delta)/r_b/MATLAB Function ==
  data: r_ref input; r output; T_ref input; T input; alpha input
function r = thermalResistance(r_ref, T_ref, T, alpha)

r = r_ref * (1 + alpha * (T - T_ref));

end

== matlab function LundellAlternatorAC/Alternator/Armature circuit/Armature circuit (Delta)/r_a/MATLAB Function ==
  data: r_ref input; r output; T_ref input; T input; alpha input
function r = thermalResistance(r_ref, T_ref, T, alpha)

r = r_ref * (1 + alpha * (T - T_ref));

end

== matlab function LundellAlternatorAC/Alternator/Armature circuit/Armature circuit (Delta)/r_c/MATLAB Function ==
  data: r_ref input; r output; T_ref input; T input; alpha input
function r = thermalResistance(r_ref, T_ref, T, alpha)

r = r_ref * (1 + alpha * (T - T_ref));

end

== matlab function LundellAlternatorAC/Alternator/Armature circuit/Armature circuit (Y)/r_a/MATLAB Function ==
  data: r_ref input; r output; T_ref input; T input; alpha input
function r = thermalResistance(r_ref, T_ref, T, alpha)

r = r_ref * (1 + alpha * (T - T_ref));

end

== matlab function LundellAlternatorAC/Alternator/Armature circuit/Armature circuit (Y)/r_b/MATLAB Function ==
  data: r_ref input; r output; T_ref input; T input; alpha input
function r = thermalResistance(r_ref, T_ref, T, alpha)

r = r_ref * (1 + alpha * (T - T_ref));

end

== matlab function LundellAlternatorAC/Alternator/Armature circuit/Armature circuit (Y)/r_c/MATLAB Function ==
  data: r_ref input; r output; T_ref input; T input; alpha input
function r = thermalResistance(r_ref, T_ref, T, alpha)

r = r_ref * (1 + alpha * (T - T_ref));

end
